simulink model "IMU_board_example"  (R2015b)
settings: Solver=ode1  StartTime=0.0  StopTime=inf  FixedStep=.0005  RelTol=1e-3
undefined symbols (not defined in the file): deg, s
libraries: qbmove_library x2, qbmove_library_2015b x1, QB_pacer_lib x1
settings Model: Creator=laurentio  LastModifiedBy=MattiaCP
settings DataIOCC: SaveFormat=Array
settings DebuggingCC: UnderspecifiedInitializationDetection=Classic  MergeDetectMultiDrivingBlocksExec=none  SolverPrmCheckMsg=warning  StateNameClashWarn=warning
settings HardwareCC: ProdBitPerPointer=32  ProdLargestAtomicFloat=None  ProdIntDivRoundTo=Undefined  ProdEndianess=Unspecified  ProdWordSize=32  ProdHWDeviceType=32-bit Generic
settings GRTTargetCC: GeneratePreprocessorConditionals=Disable all
settings ConfigComp: CovModelRefEnable=Off  CovSFcnEnable=off

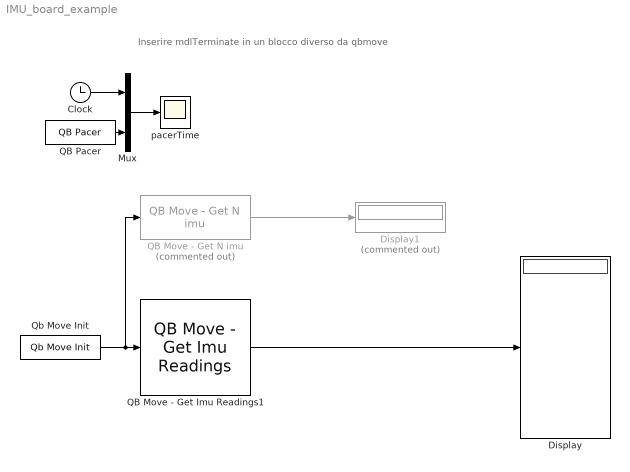
== system IMU_board_example ==
  note: Inserire mdlTerminate in un blocco diverso da qbmove
  Clock : Clock
  Display : Display
  Display1 : Display  Commented=on
  Mux : Mux  Inputs=2
  QB Move - Get Imu Readings1 : qbmove_library/QB Move - Get Imu Readings  ID=1  N_IMU=1  DAISY_CHAINING=off  ACC_SF=0.000122  GYRO_SF=0.061037  MAG_SF=0.1465  ACC_UNITY=G  GYRO_UNITY=deg/s  MAG_UNITY=uT  id0=0  acc0=on  gyro0=on  mag0=on  id1=1  acc1=on  gyro1=on  mag1=off  id2=2  acc2=on  gyro2=on  mag2=off  id3=3  acc3=on  gyro3=on  mag3=off  id4=12  acc4=on  gyro4=on  mag4=off  id5=15  acc5=on  gyro5=on  mag5=off  id6=0  acc6=on  gyro6=on  mag6=off  id7=0  acc7=on  gyro7=on  mag7=off  id8=0  acc8=on  gyro8=on  mag8=off  id9=0  acc9=on  gyro9=on  mag9=off  id10=0  acc10=on  gyro10=on  mag10=off  id11=0  acc11=on  gyro11=on  mag11=off  id12=0  acc12=on  gyro12=on  mag12=off  id13=0  acc13=on  gyro13=on  mag13=off  id14=0  acc14=on  gyro14=on  mag14=off  id15=0  acc15=on  gyro15=on  mag15=off  id16=0  acc16=on  gyro16=on  mag16=off
  QB Move - Get N imu : qbmove_library_2015b/QB Move - Get N imu  Commented=on  ID=1  CONTROL_MODE=Prime Movers Positions  DAISY_CHAINING=off
  QB Pacer : QB_pacer_lib/QB Pacer  simTimePerRealTime=1
  Qb Move Init : qbmove_library/Qb Move Init  NUMBER_OF_COM='COM2'  BAUD_RATE_COM=2000000
  pacerTime : Scope
  wires:
  QB Pacer/1 -> Mux/2
  Clock/1 -> Mux/1
  Qb Move Init/1 -> QB Move - Get N imu/1, QB Move - Get Imu Readings1/1
  Mux/1 -> pacerTime/1
  QB Move - Get Imu Readings1/1 -> Display/1
  QB Move - Get N imu/1 -> Display1/1
